simulink model "ErroAtuanteRegime"  (R2022b)
settings: Solver=ode45  StartTime=0.0  StopTime=20  RelTol=1e-6  EnableMultiTasking=on
values from neighbouring files (symbols this model uses):
  Ki = -K(3)    [PrPara2nl_PI.m]    (also in TestesEEcanalI.m = -Ka(4),K=Ka(1:3),; para2nl_PI.m)
  Kp = -Ki/p    [PrPara2nl_PI.m]    (also in para2nl_PI.m)
libraries: simulink x2
settings Model: Creator=adolfobs  LastModifiedBy=adolfo
settings SolverCC: AlgebraicLoopSolver=TrustRegion
settings DataIOCC: LimitDataPoints=on  SaveFormat=Array  SignalLoggingSaveFormat=ModelDataLogs  ReturnWorkspaceOutputs=off
settings OptimizationCC: InitFltsAndDblsToZero=on  LifeSpan=inf
settings DebuggingCC: SaveWithParameterizedLinksMsg=none  UnderspecifiedInitializationDetection=Classic  MergeDetectMultiDrivingBlocksExec=none  SignalResolutionControl=TryResolveAllWithWarning  SolverPrmCheckMsg=warning  MultiTaskDSMMsg=warning  MultiTaskCondExecSysMsg=none  UnconnectedInputMsg=warning  UnconnectedOutputMsg=warning  UnconnectedLineMsg=warning  StateNameClashWarn=warning  SFUnexpectedBacktrackingDiag=warning  SFNoUnconditionalDefaultTransitionDiag=warning  SFExecutionAtInitializationDiag=none  SFMachineParentedDataDiag=warning  ArithmeticOperatorsInVariantConditions=warning
settings HardwareCC: ProdBitPerPointer=32  ProdBitPerSizeT=32  ProdBitPerPtrDiffT=32  ProdLargestAtomicFloat=None  ProdIntDivRoundTo=Undefined  ProdEndianess=Unspecified  ProdWordSize=32  ProdHWDeviceType=32-bit Generic
settings ModelReferenceCC: EnableRefExpFcnMdlSchedulingChecks=on  PropagateSignalLabelsOutOfModel=off
settings SFSimCC: SimUseLocalCustomCode=off  CustomCodeUndefinedFunction=UseInterfaceOnly
settings RTWCC: RTWUseLocalCustomCode=off
settings CodeAppCC: StateflowObjectComments=on
settings GRTTargetCC: TargetFcnLib=ansi_tfl_tmw.mat  TargetLangStandard=C89/C90 (ANSI)  CombineOutputUpdateFcns=off  GRTInterface=on
settings ConfigComp: CovMetricSettings=dw  CovSaveCumulativeToWorkspaceVar=on  CovSaveSingleToWorkspaceVar=on  CovExternalEMLEnable=off

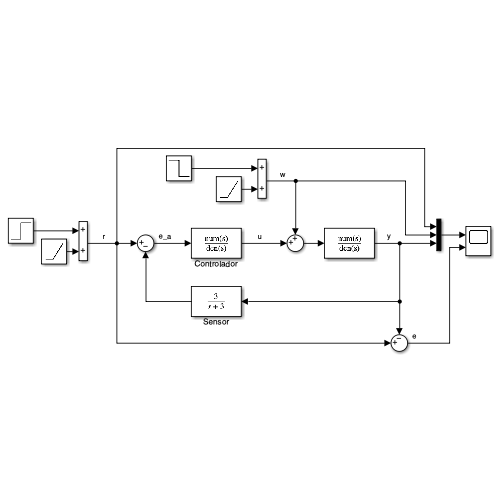
[thumbnail: Simulink's stored preview of the top-level diagram]
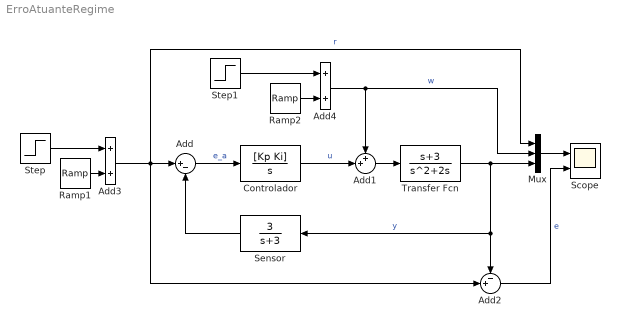
== system ErroAtuanteRegime ==
  Add : Sum  Inputs=|+-
  Add1 : Sum  Inputs=++|
  Add2 : Sum  Inputs=-+|
  Add3 : Sum
  Add4 : Sum
  Controlador : TransferFcn  Numerator=[Kp Ki]  Denominator=[1 0]
  Mux : Mux  Inputs=3
  Ramp1 : simulink/Sources/Ramp  slope=1  start=5  InitialOutput=0
  Ramp2 : simulink/Sources/Ramp  slope=1  start=15  InitialOutput=0
  Scope : Scope  NumInputPorts=2
  Sensor : TransferFcn  Numerator=[3]  Denominator=[1 3]
  Step : Step  SampleTime=0
  Step1 : Step  Time=10  After=-1  SampleTime=0
  Transfer Fcn : TransferFcn  Numerator=[1 3]  Denominator=[1 2 0]
  wires:
  Add3/1 -> Mux/1, Add2/2, Add/1  "r"
  Transfer Fcn/1 -> Add2/1, Sensor/1, Mux/3  "y"
  Add/1 -> Controlador/1  "e_a"
  Mux/1 -> Scope/1
  Add2/1 -> Scope/2  "e"
  Sensor/1 -> Add/2
  Add1/1 -> Transfer Fcn/1
  Controlador/1 -> Add1/2  "u"
  Step/1 -> Add3/1
  Ramp1/1 -> Add3/2
  Step1/1 -> Add4/1
  Ramp2/1 -> Add4/2
  Add4/1 -> Add1/1, Mux/2  "w"
